simulink model "simexa31"  (Simulink 4.00)
settings: Solver=ode23  SolverMode=SingleTasking  StartTime=0.0  StopTime=20  MaxStep=0.1  RelTol=1e-3  AbsTol=1e-3
settings Model: LastModifiedBy=saadat  SaveTime=off  SaveOutput=off  LimitDataPoints=off  RTWTemplateMakefile=grt_vc.tmf  ExtModeTrigMode=oneshot  ExtModeArmWhenConnect=off

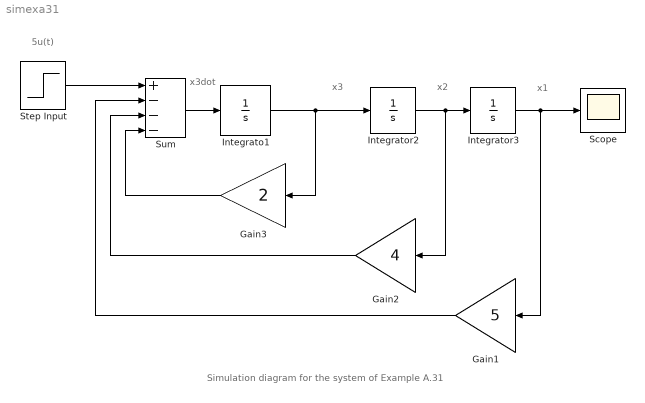
== system simexa31 ==
  note: Simulation diagram for the system of Example A.31
  note: x3
  note: x2
  note: x1
  note: x3dot
  note: 5u(t)
  Gain1 : Gain  Orientation=left  Gain=5  Multiplication=Element-wise(K.*u)  SaturateOnIntegerOverflow=on
  Gain2 : Gain  Orientation=left  Gain=4  Multiplication=Element-wise(K.*u)  SaturateOnIntegerOverflow=on
  Gain3 : Gain  Orientation=left  Gain=2  Multiplication=Element-wise(K.*u)  SaturateOnIntegerOverflow=on
  Integrato1 : Integrator  ExternalReset=none  InitialConditionSource=internal  InitialCondition=0  LimitOutput=off  UpperSaturationLimit=inf  LowerSaturationLimit=-inf  ShowSaturationPort=off  ShowStatePort=off  AbsoluteTolerance=auto
  Integrator2 : Integrator  ExternalReset=none  InitialConditionSource=internal  InitialCondition=0  LimitOutput=off  UpperSaturationLimit=inf  LowerSaturationLimit=-inf  ShowSaturationPort=off  ShowStatePort=off  AbsoluteTolerance=auto
  Integrator3 : Integrator  ExternalReset=none  InitialConditionSource=internal  InitialCondition=0  LimitOutput=off  UpperSaturationLimit=inf  LowerSaturationLimit=-inf  ShowSaturationPort=off  ShowStatePort=off  AbsoluteTolerance=auto
  Scope : Scope
      settings: TickLabels=on  TimeRange=auto  YMin=-5  YMax=5  SaveToWorkspace=off  SaveName=ScopeData  DataFormat=Array  LimitDataPoints=on  MaxDataPoints=5000
  Step Input : Step  Time=0  Before=0  After=5  SampleTime=0
  Sum : Sum  Inputs=+---  SaturateOnIntegerOverflow=on
  wires:
  Step Input/1 -> Sum/1
  Sum/1 -> Integrato1/1
  Integrato1/1 -> Integrator2/1, Gain3/1
  Gain3/1 -> Sum/4
  Gain2/1 -> Sum/3
  Gain1/1 -> Sum/2
  Integrator2/1 -> Integrator3/1, Gain2/1
  Integrator3/1 -> Scope/1, Gain1/1
